simulink model "InvertedPend_v3"  (Simulink 8.7)
settings: Solver=VariableStepAuto  StartTime=0.0  StopTime=1000  FixedStep=0.1  MaxStep=1e-3  RelTol=1e-3
values from neighbouring files (symbols this model uses):
  J = 1e-6    (= 1e-06)    [constants.m]    (also in pendulum.m)
  K = lqr( sys_ss , diag ( [ 10 1 100 1 ] ) , 1)    [pendulum.m]
  L = 0.2    [constants.m]    (also in pendulum.m)
  m = 0.1    [constants.m]    (also in pendulum.m)
  r = 50e-3    (= 0.05)    [constants.m]    (also in pendulum.m)
undefined symbols (not defined in the file): M, step_time
settings Model: Creator=Patrick  LastModifiedBy=WadeJensen
settings DataIOCC: SignalLoggingSaveFormat=ModelDataLogs
settings OptimizationCC: ExpressionDepthLimit=2147483647
settings DebuggingCC: SolverPrmCheckMsg=warning  FcnCallInpInsideContextMsg=EnableAllAsWarning  StateNameClashWarn=warning
settings GRTTargetCC: CombineOutputUpdateFcns=off  GRTInterface=on

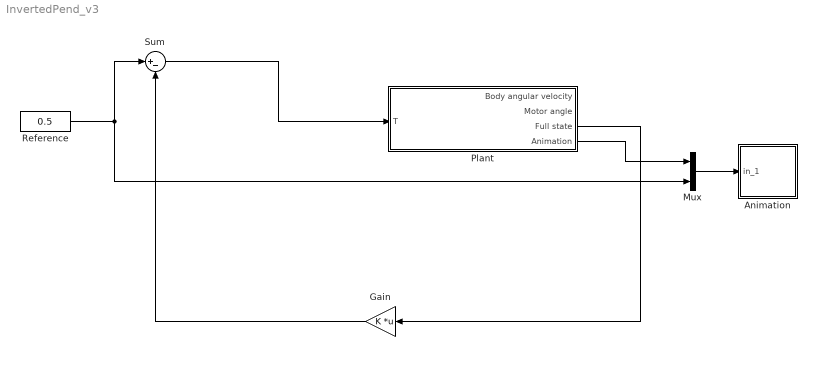
== system InvertedPend_v3 ==
  Animation : Subsystem  mask(Pendulum plot){RefBlock=Reference, L=L, r=r, Ts=step_time}
      mask prompts: RefBlock "DC reference signal block name:"; L "Location of mass"; r "Radius of wheel"; Ts "Simulation time step"
      mask help: Pendulum plot
      mask Help: Pendulum animation function using Handle graphics.
      mask Display: plot([-10 10],[0 0],[-2 -2 2 2],[0 1 1 0],[0 3],[1 5])
  Gain : Gain  Gain=K  Multiplication=Matrix(K*u)
  Mux : Mux  Inputs=2
  Plant : Subsystem  mask{m=m, mw=M, J=J, r=r, L=L, g=9.81, theta0=0.1}
      mask prompts: m "Mass of body"; mw "Mass of wheel"; J "Inertia of wheel"; r "Radius of wheel"; L "Height of body COM"; g "Gravity"; theta0 "Initial angle"
  Reference : Constant  Value=0.5
  Sum : Sum  Inputs=|+-
  wires:
  Mux/1 -> Animation/1(in_1)
  Plant/4(Animation) -> Mux/1
  Reference/1 -> Mux/2, Sum/1
  Sum/1 -> Plant/1(T)
  Plant/3(Full state) -> Gain/1
  Gain/1 -> Sum/2

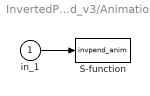
== system InvertedPend_v3/Animation ==
  in_1 : Inport
  S-function : S-Function  FunctionName=invpend_anim  Parameters=RefBlock,L,r,Ts  SFunctionDeploymentMode=off  EnableBusSupport=off
      settings: DeleteFcn=pendan([],[],[],'DeleteBlock');
  wires:
  in_1/1 -> S-function/1

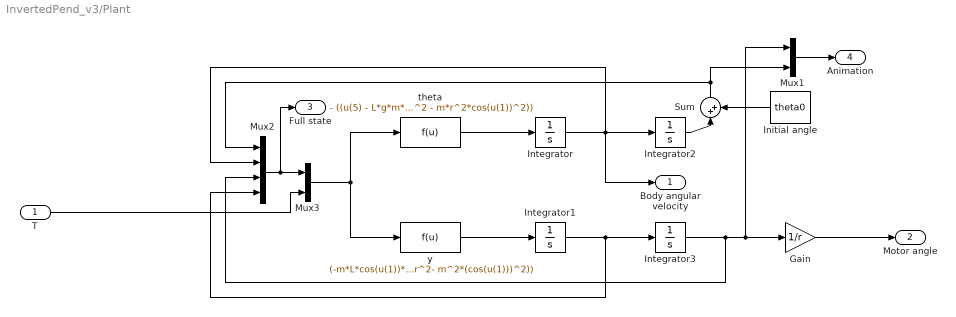
== system InvertedPend_v3/Plant ==
  T : Inport
  Gain : Gain  Gain=1/r
  Initial angle : Constant  Value=theta0
  Integrator{,1..3} (4 alike) : Integrator
  Mux1 : Mux  Inputs=2
  Mux2 : Mux
  Mux3 : Mux  Inputs=2
  Sum : Sum  Inputs=|++
  theta : Fcn  Expr=- ((u(5) - L*g*m*sin(u(1)))*(J + m*r^2 + mw*r^2))/(L^2*m*(J + m*r^2 + mw*r^2 - m*r^2*cos(u(1))^2)) - (r^2*cos(u(1))*(u(5)/r + L*m*u(2)^2*sin(u(1))))/(L*(J + m*r^2 + mw*r^2 - m*r^2*cos(u(1))^2))
  y : Fcn  Expr=(-m*L*cos(u(1))*(m*g*L*sin(u(1)) - u(5)) + m*L^2*(m*L*u(2)^2*sin(u(1))+u(5)/r))/(L^2*(m^2+m*mw+(m*J)/r^2- m^2*(cos(u(1)))^2))
  Body angular velocity : Outport
  Motor angle : Outport  Port=2
  Full state : Outport  Port=3
  Animation : Outport  Port=4
  wires:
  theta/1 -> Integrator/1
  y/1 -> Integrator1/1
  Integrator/1 -> Body angular velocity/1, Integrator2/1, Mux2/2
  Integrator1/1 -> Integrator3/1, Mux2/4
  Integrator3/1 -> Gain/1, Mux1/1, Mux2/3
  T/1 -> Mux3/2
  Gain/1 -> Motor angle/1
  Integrator2/1 -> Sum/1
  Sum/1 -> Mux1/2, Mux2/1
  Initial angle/1 -> Sum/2
  Mux1/1 -> Animation/1
  Mux2/1 -> Mux3/1, Full state/1
  Mux3/1 -> theta/1, y/1
